simulink model "l1_soft_sil"  (R2026a)
settings: Solver=FixedStepDiscrete  StopTime=t_final  FixedStep=dt_sim
PreLoadFcn:
  | run('l1_init.m')
libraries: l1_blocks x6
settings Model: Creator=eduno  LastModifiedBy=eduno

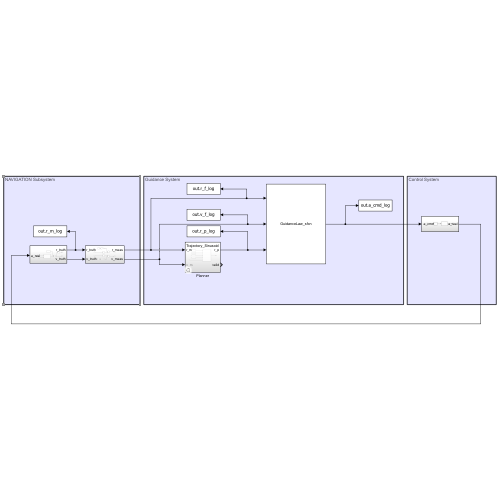
[thumbnail: Simulink's stored preview of the top-level diagram]
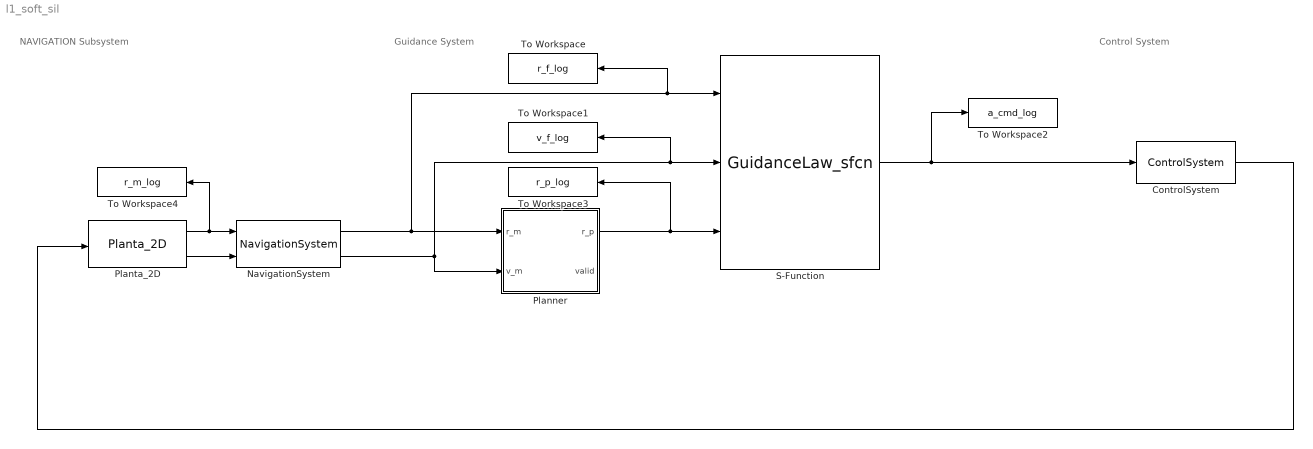
== system l1_soft_sil ==
  note: Control System
  note: NAVIGATION Subsystem
  note: Guidance System
  ControlSystem : l1_blocks/ControlSystem  SystemSampleTime=-1  VariantActivationTime=update diagram  EmptyChoice=off  PassThrough=off  PassThroughVariantControl=(default)  EmptyChoiceVariantControl=(default)  AllowFlexibleInterface=on  Latency=0  AutoFrameSizeCalculation=off
  NavigationSystem : l1_blocks/NavigationSystem  SystemSampleTime=-1  VariantActivationTime=update diagram  EmptyChoice=off  PassThrough=off  PassThroughVariantControl=(default)  EmptyChoiceVariantControl=(default)  AllowFlexibleInterface=on  Latency=0  AutoFrameSizeCalculation=off
  Planner : Subsystem  Variant=on
  Planta_2D : l1_blocks/Planta_2D  SystemSampleTime=-1  VariantActivationTime=update diagram  EmptyChoice=off  PassThrough=off  PassThroughVariantControl=(default)  EmptyChoiceVariantControl=(default)  AllowFlexibleInterface=on  Latency=0  AutoFrameSizeCalculation=off
  S-Function : S-Function  FunctionName=GuidanceLaw_sfcn  SFunctionDeploymentMode=off  EnableBusSupport=off
  To Workspace : ToWorkspace  VariableName=r_f_log  SaveFormat=Timeseries  SampleTime=-1
  To Workspace1 : ToWorkspace  VariableName=v_f_log  SaveFormat=Timeseries  SampleTime=-1
  To Workspace2 : ToWorkspace  VariableName=a_cmd_log  SaveFormat=Timeseries  SampleTime=-1
  To Workspace3 : ToWorkspace  VariableName=r_p_log  SaveFormat=Timeseries  SampleTime=-1
  To Workspace4 : ToWorkspace  VariableName=r_m_log  SaveFormat=Timeseries  SampleTime=-1
  wires:
  NavigationSystem/1 -> S-Function/1, To Workspace/1, Planner/1(r_m)
  NavigationSystem/2 -> Planner/2(v_m), S-Function/2, To Workspace1/1
  S-Function/1 -> ControlSystem/1, To Workspace2/1
  Planner/1(r_p) -> S-Function/3, To Workspace3/1
  ControlSystem/1 -> Planta_2D/1
  Planta_2D/1 -> To Workspace4/1, NavigationSystem/1
  Planta_2D/2 -> NavigationSystem/2

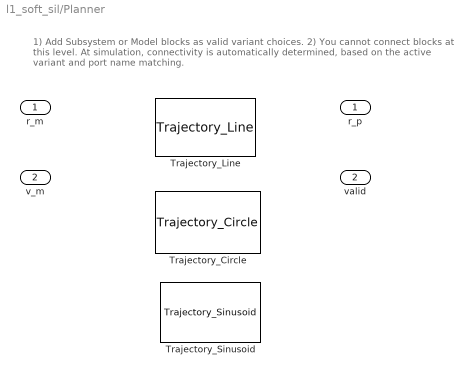
== system l1_soft_sil/Planner ==
  note: 1) Add Subsystem or Model blocks as valid variant choices.
      | 2) You cannot connect blocks at this level. At simulation, connectivity is automatically
      | determined, based on the active variant and port name matching.
  r_m : Inport
  v_m : Inport  Port=2
  Trajectory_Circle : l1_blocks/Trajectory_Circle  SystemSampleTime=-1  VariantControl=VAR_CIRCLE  VariantActivationTime=update diagram  EmptyChoice=off  PassThrough=off  PassThroughVariantControl=(default)  EmptyChoiceVariantControl=(default)  AllowFlexibleInterface=on  Latency=0  AutoFrameSizeCalculation=off
  Trajectory_Line : l1_blocks/Trajectory_Line  SystemSampleTime=-1  VariantControl=VAR_LINE  VariantActivationTime=update diagram  EmptyChoice=off  PassThrough=off  PassThroughVariantControl=(default)  EmptyChoiceVariantControl=(default)  AllowFlexibleInterface=on  Latency=0  AutoFrameSizeCalculation=off
  Trajectory_Sinusoid : l1_blocks/Trajectory_Sinusoid  SystemSampleTime=-1  VariantControl=VAR_SINUSOID  VariantActivationTime=update diagram  EmptyChoice=off  PassThrough=off  PassThroughVariantControl=(default)  EmptyChoiceVariantControl=(default)  AllowFlexibleInterface=on  Latency=0  AutoFrameSizeCalculation=off
  r_p : Outport
  valid : Outport  Port=2
